simulink model "motor_io"  (Simulink 8.4)
settings: Solver=ode1  StartTime=0.0  StopTime=inf  FixedStep=Ts  RelTol=1e-3
PostLoadFcn:
  | , if any(exist('dsrtsu_mdlpostloadfcn', 'file') == [2, 3, 6]), try dsrtsu_mdlpostloadfcn('Execute', bdroot); catch fprintf('Error in PostLoadFcn (dsrtsu_mdlpostloadfcn) for model "%s":\n %s\n', bdroot, lasterr); end, end,
values from neighbouring files (symbols this model uses):
  enable_karnop = 1    [workshop1.m]
  F_c = 1e-3    (= 0.001)    [workshop1.m]
  J = J1+J2    (= 3.6e-05)    [workshop1.m]
  Jtot = motor.J + J/n^2    [workshop1.m]
  motor = motor_pars    [workshop1.m]
  n = 5    [workshop1.m]
  Ts = 0.02    [workshop1.m]
libraries: rtilib1104 x5, simulink x1
settings Model: DSRTSU_INTERNAL_RTI_VER=450  DSRTSU_INTERNAL_RTI_TYPE=rti1104  DSRTSU_INTERNAL_RTIFPGA=40  Creator=user  LastModifiedBy=es2lab2  ExtModeArmWhenConnect=off  BufferReuse=off
settings DataIOCC: SaveOutput=off  SignalLoggingName=sigsOut
settings OptimizationCC: BlockReduction=off  ConditionallyExecuteInputs=off  OptimizeBlockIOStorage=off  BufferReuse=off  GlobalBufferReuse=off  ExpressionFolding=off  LocalBlockOutputs=off  InitFltsAndDblsToZero=on
settings DebuggingCC: SaveWithParameterizedLinksMsg=none  SignalResolutionControl=TryResolveAllWithWarning  SolverPrmCheckMsg=none  MultiTaskDSMMsg=warning  MultiTaskCondExecSysMsg=none  UnconnectedInputMsg=none  UnconnectedOutputMsg=none
settings HardwareCC: ProdIntDivRoundTo=Zero  ProdEndianess=BigEndian  ProdHWDeviceType=Generic->Custom  TargetIntDivRoundTo=Zero  TargetEndianess=BigEndian  TargetHWDeviceType=Generic->Custom
settings RTWCC: SystemTargetFile=rti1104.tlc  MakeCommand=make_rti  TemplateMakefile=rti1104.tmf  Description=dSPACE DS1104 Hardware Platform  RetainRTWFile=on  ProcessScript=rti1104_make_rtw_hook  IncludeERTFirstTime=on
settings STFCustomTargetCC: TargetFcnLib=ansi_tfl_tmw.mat  ParMdlRefBuildCompliant=on  GeneratePreprocessorConditionals=Disable all  SystemTargetFile=rti1104.tlc
settings GRTTargetCC: TargetFcnLib=ansi_tfl_tmw.mat  CompOptLevelCompliant=off  ConcurrentExecutionCompliant=off  MatFileLogging=off  CPPClassGenCompliant=off  ExtModeMexFile=noextcomm
settings CustomProperty: DataType=RTWOptions_EnumType_C__Program Files (x86)_dSPACE RCPHIL 2014-B_MATLAB_RTI_RTI1104_TLC_rti1104_1InitialSimState  Value=RUN
settings EnumStrPairs: String=RUN

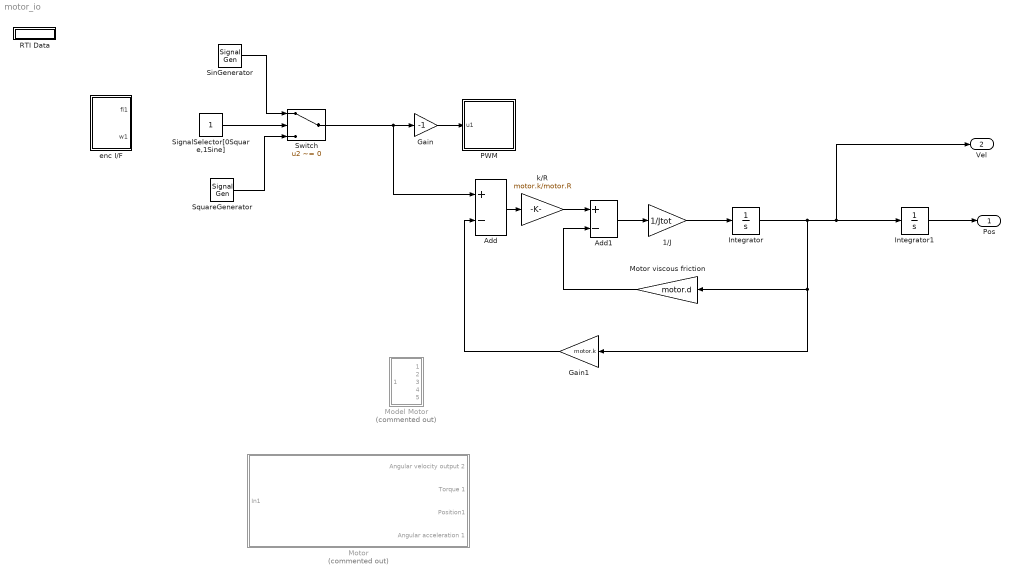
== system motor_io ==
  1/J : Gain  Gain=1/Jtot
  Add : Sum  Inputs=+-
  Add1 : Sum  Inputs=+-
  Gain : Gain  Gain=-1
  Gain1 : Gain  Gain=motor.k
  Integrator : Integrator
  Integrator1 : Integrator
  Model Motor : Subsystem  Commented=on
  Motor : Subsystem  Commented=on
  Motor viscous friction : Gain  Gain=motor.d
  PWM : Subsystem
  RTI Data : Subsystem  Tag=struct('RTIDataServer',struct('RTIDataServerVs','2','RTIModelDescription','struct(''main'',''motor_io'',''sub'','''',''isMp'',0)'))  LoadFcn="if exist('rtidc'), try,  rtidc('DataHostBlockClbLoad', gcbh); catch, disp(['Warning: ''LoadFcn'' for RTI Data block failed: ' lasterr]); end, end,"  mask(RTI_DATA_HOST){}
      mask help:
      | RTI Data Block.
      | This block is used by RTI to store internal model-dependent data.
      | Please keep this block on the root level of the model. Deleting this block will result in data loss.
      |
      | NEVER DELETE OR COPY THIS BLOCK!
      settings: CopyFcn="if exist('rtidc'), try,  rtidc('DataHostBlockClbCopy', gcbh); catch, disp(['Warning: ''CopyFcn'' for RTI Data block failed: ' lasterr]); end, end,"  DeleteFcn="if exist('rtidc'), try,  rtidc('DataHostBlockClbDelete', gcbh); catch, disp(['Warning: ''DeleteFcn'' for RTI Data block failed: ' lasterr]); end, end,"  ModelCloseFcn="if exist('rtidc'), try,  rtidc('DataHostBlockClbModelClose', gcbh); catch, disp(['Warning: ''ModelCloseFcn'' for RTI Data block failed: ' lasterr]); end, end,"  PreSaveFcn="if exist('rtidc'), try,  rtidc('DataHostBlockClbPreSave', gcbh); catch, disp(['Warning: ''PreSaveFcn'' for RTI Data block failed: ' lasterr]); end, end,"  PostSaveFcn="if exist('rtidc'), try,  rtidc('DataHostBlockClbPostSave', gcbh); catch, disp(['Warning: ''PostSaveFcn'' for RTI Data block failed: ' lasterr]); end, end,"  NameChangeFcn="if exist('rtidc'), try,  rtidc('DataHostBlockClbNameChange', gcbh); catch, disp(['Warning: ''NameChangeFcn'' for RTI Data block failed: ' lasterr]); end, end,"
      mask Help:
      | RTI Data Block.
      | This block is used by RTI to store internal model-dependent data.
      | Please keep this block on the root level of the model. Deleting this block will result in data loss.
      | 
      | NEVER DELETE OR COPY THIS BLOCK!
      mask Display:
      | text(0.5, 0.5, 'RTI Data', 'HorizontalAlignment', 'center');
      | plot([1 0]);
  SignalSelector[0Square,1Sine] : Constant
  SinGenerator : SignalGenerator  Amplitude=0  Units=rad/sec
  SquareGenerator : SignalGenerator  WaveForm=square  Amplitude=0  Units=rad/sec
  Switch : Switch  Criteria=u2 ~= 0
  enc I/F : Subsystem
  "k/R " : Gain  Gain=motor.k/motor.R
  Pos : Outport
  Vel : Outport  Port=2
  wires:
  SinGenerator/1 -> Switch/1
  SquareGenerator/1 -> Switch/3
  SignalSelector[0Square,1Sine]/1 -> Switch/2
  Switch/1 -> Add/1, Gain/1
  Gain1/1 -> Add/2
  Add/1 -> "k/R "/1
  "k/R "/1 -> Add1/1
  Add1/1 -> 1/J/1
  1/J/1 -> Integrator/1
  Integrator/1 -> Motor viscous friction/1, Gain1/1, Vel/1, Integrator1/1
  Motor viscous friction/1 -> Add1/2
  Integrator1/1 -> Pos/1
  Gain/1 -> PWM/1(u1)

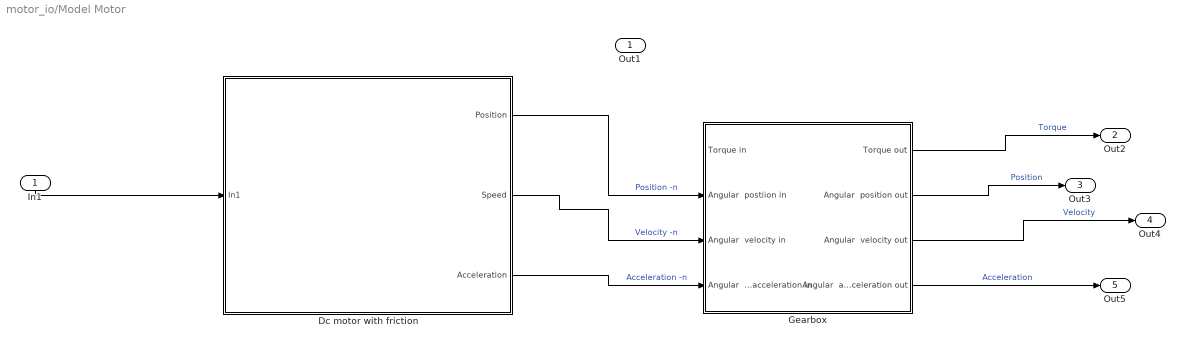
== system motor_io/Model Motor ==
  In1 : Inport
  Dc motor with friction : Subsystem
      mask Display:
      | image('dcmotor.jpg')
      | port_label('input', 1, 'Voltage')
      | port_label('output', 1, 'Current')
      | port_label('output', 2, 'Torque')
      | port_label('output', 3, 'Position')
      | port_label('output', 4, 'Velocity')
      | port_label('output', 5, 'Acceleration')
  Gearbox : Subsystem
  Out1 : Outport
  Out2 : Outport  Port=2
  Out3 : Outport  Port=3
  Out4 : Outport  Port=4
  Out5 : Outport  Port=5
  wires:
  Dc motor with friction/2(Speed) -> Gearbox/3(Angular  velocity in)  "Velocity -n"
  ? -> Gearbox/1(Torque in)  "Torque -n"
  Dc motor with friction/3(Acceleration) -> Gearbox/4(Angular  acceleration in)  "Acceleration -n"
  Dc motor with friction/1(Position) -> Gearbox/2(Angular  postiion in)  "Position -n"
  In1/1 -> Dc motor with friction/1(In1)
  Gearbox/1(Torque out) -> Out2/1  "Torque"
  ? -> Out1/1  "Current"
  Gearbox/2(Angular  position out) -> Out3/1  "Position"
  Gearbox/4(Angular  acceleration out) -> Out5/1  "Acceleration"
  Gearbox/3(Angular  velocity out) -> Out4/1  "Velocity"

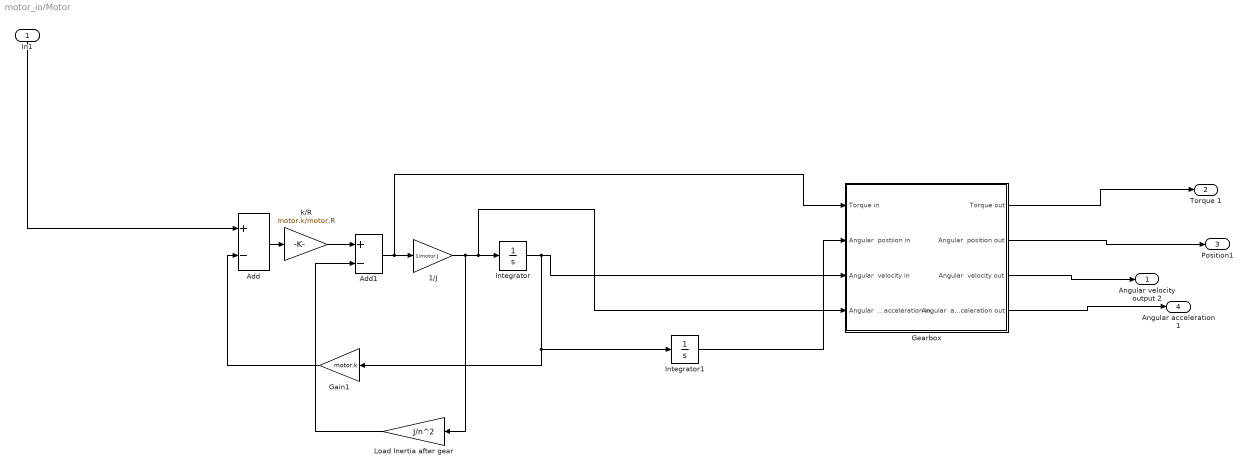
== system motor_io/Motor ==
  In1 : Inport
  1/J : Gain  Gain=1/motor.J
  Add : Sum  Inputs=+-
  Add1 : Sum  Inputs=+-
  Gain1 : Gain  Gain=motor.k
  Gearbox : Subsystem
  Integrator : Integrator
  Integrator1 : Integrator
  Load Inertia after gear : Gain  Gain=J/n^2
  "k/R " : Gain  Gain=motor.k/motor.R
  Angular velocity output 2 : Outport
  Torque 1 : Outport  Port=2
  Position1 : Outport  Port=3
  Angular acceleration 1 : Outport  Port=4
  wires:
  Integrator1/1 -> Gearbox/2(Angular  postiion in)
  Add/1 -> "k/R "/1
  "k/R "/1 -> Add1/1
  1/J/1 -> Load Inertia after gear/1, Gearbox/4(Angular  acceleration in), Integrator/1
  Add1/1 -> Gearbox/1(Torque in), 1/J/1
  Gain1/1 -> Add/2
  Integrator/1 -> Gearbox/3(Angular  velocity in), Integrator1/1, Gain1/1
  In1/1 -> Add/1
  Gearbox/4(Angular  acceleration out) -> Angular acceleration 1/1
  Gearbox/3(Angular  velocity out) -> Angular velocity output 2/1
  Gearbox/2(Angular  position out) -> Position1/1
  Gearbox/1(Torque out) -> Torque 1/1
  Load Inertia after gear/1 -> Add1/2

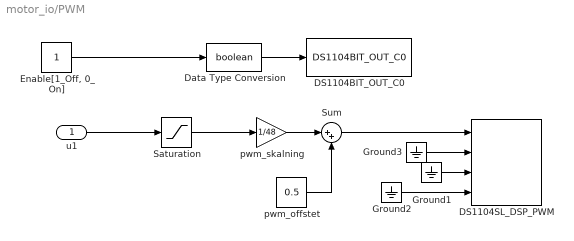
== system motor_io/PWM ==
  u1 : Inport
  DS1104BIT_OUT_C0 : rtilib1104/DS1104 MASTER PPC/DS1104BIT_OUT_C0  ChannelNo=0  InitValue=1  TermMode=0  TermValue=0  Reserved1=[]  Reserved2=[]  Reserved3=[]  Reserved=[]  DialogFcn=gui1104bit_out  UnitName={'DS1104BIT_OUT_C'}  UnitValues={ 0 }  DSProperties=struct('RTI',struct('Version',uint32(1),'BlockType',struct('isSLSource',uint8(0),'isSLSink',uint8(1),'isHWSource',uint8(0),'isHWSink',uint8(1),'isSetup',uint8(0),'isInline',uint8(1),'isNonInline',uint8(0),'isInterrupt',uint8(0),'isChannelwise',uint8(1)),'IOBoardType','DS1104MASTER','UnitType','BIT','Identifier','BITOUTCH','DialogType','ML','BlockSet','NONE','SlaveProcessor','NONE'))
  DS1104SL_DSP_PWM : rtilib1104/DS1104 SLAVE DSP/DS1104SL_DSP_PWM  Parameters=[]  TDef=[]  BoardType=[]  PwmMode=1  Frequency=20000  InitValue=[0.5 0.5 0.5 0.5]  TermMode=[0 0 0 0]  TermValue=[0.5 0.5 0.5 0.5]  Polarity=[1 1 1 1]  DialogFcn=gui1104sl_dsp_pwm  Reserved1=[]  Reserved2=[]  Reserved3=[]  Reserved4=[]  Revision=[]  UnitName={'DS1104SL_DSP_PWM'}  UnitValues={[]}  DSProperties=struct('RTI',struct('Version',uint32(2),'BlockType',struct('isSLSource',uint8(0),'isSLSink',uint8(1),'isHWSource',uint8(0),'isHWSink',uint8(1),'isSetup',uint8(0),'isInline',uint8(1),'isNonInline',uint8(0),'isInterrupt',uint8(0),'isChannelwise',uint8(0)),'IOBoardType','DS1104SLAVE','UnitType','PWM','Identifier','PWM','DialogType','ML','BlockSet','NONE','SlaveProcessor','F240'))  RTIBlockInterface=struct('InputPortsActive',[1 1 1 1],'InputPortsWidth',int32([1 1 1 1]),'InputPortsName',{{['PWM Channel 1'],['PWM Channel 2'],['PWM Channel 3'],['PWM Channel 4']}},'IWork',{{{'',uint32(4)}}},'DialogFcn','rti1104slavepwmgui','InitLevel',1,'BlockDisplay',{{'','auto'}},'IconTransparency','on','MultiSFcn',4,'BlockName',struct('Token',{{'DS1104SL_DSP_PWM'}}))  RTIBlockParameters=struct('PWMSymmetryMode',{{1,'OFF',[]}},'PWMFrequency',{{'50000','OFF',[]}},'PWMPolarityMode',{{[1 1 1 1 1],'OFF',[]}},'ChannelNo',{{[1 2 3 4],'OFF',[]}},'SuspendModeInit',{{[0 0 0 0 1],'OFF',[]}},'TTLModeInit',{{[2 2 2 2 2],'OFF',[]}},'DutyCycleInitValueCh1',{{'0.5','OFF',[]}},'DutyCycleInitValueCh2',{{'0.5','OFF',[]}},'DutyCycleInitValueCh3',{{'0.5','OFF',[]}},'DutyCycleInitValueCh4',{{'0.5','OFF',[]}},'DutyCycleInitValueCh5',{{'0.5','OFF',[]}},'EnablePWMStop',{{[0 0 0 0 0],'OFF',[]}},'SuspendModeTerm',{{[0 0 0 0 1],'OFF',[]}},'TTLModeTerm',{{[2 2 2 2 2],'OFF',[]}},'DutyCycleTermValueCh1',{{'0.5','OFF',[]}},'DutyCycleTermValueCh2',{{'0.5','OFF',[]}},'DutyCycleTermValueCh3',{{'0.5','OFF',[]}},'DutyCycleTermValueCh4',{{'0.5','OFF',[]}},'DutyCycleTermValueCh5',{{'0.5','OFF',[]}},'TLCFileName',{{'rti1104pwm','OFF',[]}})  RTISFcnParameters=struct('PWMSymmetryMode','double','PWMFrequency','double','PWMPolarityMode','double','ChannelNo','double','SuspendModeInit','double','TTLModeInit','double','DutyCycleInitValueCh1','double','DutyCycleInitValueCh2','double','DutyCycleInitValueCh3','double','DutyCycleInitValueCh4','double','EnablePWMStop','double','SuspendModeTerm','double','TTLModeTerm','double','DutyCycleTermValueCh1','double','DutyCycleTermValueCh2','double','DutyCycleTermValueCh3','double','DutyCycleTermValueCh4','double','TLCFileName','char')  RTIBlockParaDefault=struct('PWMSymmetryMode',1,'PWMFrequency',100,'PWMPolarityMode',[1 1 1 1 1],'ChannelNo',[1 2 3 4],'SuspendModeInit',[1 1 1 1 1],'TTLModeInit',[2 2 2 2 2],'DutyCycleInitValueCh1',0.5,'DutyCycleInitValueCh2',0.5,'DutyCycleInitValueCh3',0.5,'DutyCycleInitValueCh4',0.5,'DutyCycleInitValueCh5',0.5,'EnablePWMStop',[1 1 1 1 0],'SuspendModeTerm',[1 1 1 1 1],'TTLModeTerm',[2 2 2 2 2],'DutyCycleTermValueCh1',0.5,'DutyCycleTermValueCh2',0.5,'DutyCycleTermValueCh3',0.5,'DutyCycleTermValueCh4',0.5,'DutyCycleTermValueCh5',0.5,'TLCFileName','rti1104pwm')
  Data Type Conversion : DataTypeConversion  OutDataTypeStr=boolean  SaturateOnIntegerOverflow=on  RndMeth=Zero
  "Enable[1_Off, 0_On]" : Constant
  Ground1 : Ground
  Ground2 : Ground
  Ground3 : Ground
  Saturation : Saturate  UpperLimit=24  LowerLimit=-24
  Sum : Sum  Inputs=|++  SaturateOnIntegerOverflow=on
  pwm_offstet : Constant  Value=0.5
  pwm_skalning : Gain  Gain=1/48  SaturateOnIntegerOverflow=on  OutDataTypeStr=Inherit: Same as input  ParamDataTypeStr=Inherit: Same as input
  wires:
  "Enable[1_Off, 0_On]"/1 -> Data Type Conversion/1
  Data Type Conversion/1 -> DS1104BIT_OUT_C0/1
  pwm_skalning/1 -> Sum/1
  Sum/1 -> DS1104SL_DSP_PWM/1
  pwm_offstet/1 -> Sum/2
  u1/1 -> Saturation/1
  Ground1/1 -> DS1104SL_DSP_PWM/3
  Ground2/1 -> DS1104SL_DSP_PWM/4
  Ground3/1 -> DS1104SL_DSP_PWM/2
  Saturation/1 -> pwm_skalning/1

== system motor_io/RTI Data ==
  RTI Data Store : Subsystem  Tag="struct('public',struct('sub',struct('name',{{'motor_io'}},'data',{{struct('TH',struct('thTaskInfo',struct('taskType',{'TIMER','HWINT','TMRINT','SWINT','GLINT'},'tasksNumOf',{1,0,0,0,0},'srcIds',{{'TIMERA'},{},{},{},{}},'taskNames',{{['Timer Task 1']},{},{},{},{}})),'th_tc',struct('dataType','TASK','taskGroupId','','taskGroupList',{{}},'taskSchedulingPolicy','FCFS','taskType','TIMER','blkh',-1,'srcId','TIMERA','srcSgnName',['Timer A interrupt'],'srcCpuName','','taskName',['Timer Task 1  [0.02] s'],'taskNameDisplayExt','','smplTime',0.02,'smplTimeOffs',0,'hasFixedPriority',0,'priority',1,'hasFixedOvc',0,'ovcType',1,'ovcMax',1),'tc_th',struct('dataType','TASK','taskGroupId','','taskGroupList',{{}},'taskSchedulingPolicy','FCFS','taskType','TIMER','blkh',-1,'srcId','TIMERA','srcSgnName',['Timer A interrupt'],'srcCpuName','','taskName',['Timer Task 1  [0.02] s'],'taskNameDisplayExt','','smplTime',0.02,'smplTimeOffs',0,'hasFixedPriority',0,'priority',1,'hasFixedOvc',0,'ovcType',1,'ovcMax',1))}})),'private',struct('version',struct('dsVer',uint32(2)),'access',struct('modified',['04-Mar-2016 16:52:32'],'type','Model','isPerm',1)))"  mask(RTI_DATA_STORE){}
      mask help:
      | RTI Data Store Block. This block is used by RTI to store internal model dependent data. Deleting this block will result in data loss.
      |
      | NEVER DELETE, COPY, OR MODIFY THIS BLOCK!
      mask Help:
      | RTI Data Store Block. This block is used by RTI to store internal model dependent data. Deleting this block will result in data loss.
      | 
      | NEVER DELETE, COPY, OR MODIFY THIS BLOCK!
      mask Display: text(0.5, 0.5, ' ', 'HorizontalAlignment', 'center');

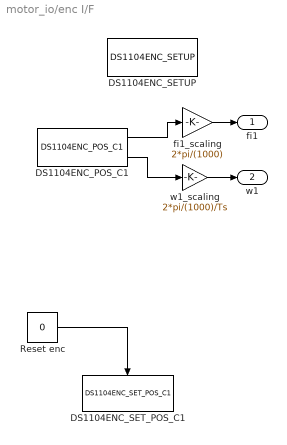
== system motor_io/enc I/F ==
  DS1104ENC_POS_C1 : rtilib1104/DS1104 MASTER PPC/DS1104ENC_POS_C1  ChannelNo=1  PosValue=0  Reserved1=[]  Reserved2=[]  Reserved3=[]  Reserved4=[]  DialogFcn=gui1104enc_pos  UnitName={'DS1104ENC_POS_C'}  UnitValues={ 1 }  DSProperties=struct('RTI',struct('Version',uint32(1),'BlockType',struct('isSLSource',uint8(1),'isSLSink',uint8(0),'isHWSource',uint8(1),'isHWSink',uint8(0),'isSetup',uint8(0),'isInline',uint8(1),'isNonInline',uint8(0),'isInterrupt',uint8(0),'isChannelwise',uint8(1)),'IOBoardType','DS1104MASTER','UnitType','ENC','Identifier','ENCPOSCH','DialogType','ML','BlockSet','NONE','SlaveProcessor','NONE'))
  DS1104ENC_SETUP : rtilib1104/DS1104 MASTER PPC/DS1104ENC_SETUP  Reserved1=[]  Reserved2=[]  Reserved3=[]  Reserved4=[]  DialogFcn=gui1104enc_setup  UnitName={'DS1104ENC_SETUP'}  UnitValues={ [] }  DSProperties=struct('RTI',struct('Version',uint32(1),'BlockType',struct('isSLSource',uint8(0),'isSLSink',uint8(0),'isHWSource',uint8(0),'isHWSink',uint8(0),'isSetup',uint8(0),'isInline',uint8(1),'isNonInline',uint8(0),'isInterrupt',uint8(0),'isChannelwise',uint8(0)),'IOBoardType','DS1104MASTER','UnitType','ENC','Identifier','ENCSETUP','DialogType','ML','BlockSet','NONE','SlaveProcessor','NONE'))
      settings: SignalType=[1 0]
  DS1104ENC_SET_POS_C1 : rtilib1104/DS1104 MASTER PPC/DS1104ENC_SET_POS_C1  ChannelNo=1  PosValue=0  Reserved1=[]  Reserved2=[]  Reserved3=[]  Reserved4=[]  DialogFcn=gui1104enc_set_pos  UnitName={'DS1104ENC_SET_POS_C'}  UnitValues={ 1 }  DSProperties=struct('RTI',struct('Version',uint32(1),'BlockType',struct('isSLSource',uint8(0),'isSLSink',uint8(1),'isHWSource',uint8(0),'isHWSink',uint8(1),'isSetup',uint8(0),'isInline',uint8(1),'isNonInline',uint8(0),'isInterrupt',uint8(0),'isChannelwise',uint8(1)),'IOBoardType','DS1104MASTER','UnitType','ENC','Identifier','ENCRESET','DialogType','ML','BlockSet','NONE','SlaveProcessor','NONE'))
  Reset enc : Constant  Value=0
  fi1_scaling : Gain  Gain=2*pi/(1000)  SaturateOnIntegerOverflow=on  OutDataTypeStr=Inherit: Same as input  ParamDataTypeStr=Inherit: Same as input
  w1_scaling : Gain  Gain=2*pi/(1000)/Ts  SaturateOnIntegerOverflow=on  OutDataTypeStr=Inherit: Same as input  ParamDataTypeStr=Inherit: Same as input
  fi1 : Outport
  w1 : Outport  Port=2
  wires:
  Reset enc/1 -> DS1104ENC_SET_POS_C1/Trigger
  DS1104ENC_POS_C1/1 -> fi1_scaling/1
  DS1104ENC_POS_C1/2 -> w1_scaling/1
  fi1_scaling/1 -> fi1/1
  w1_scaling/1 -> w1/1

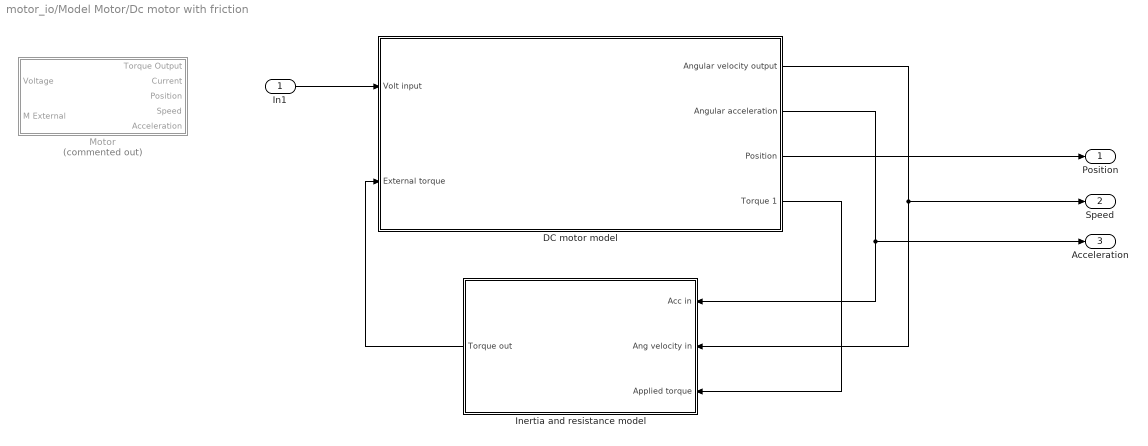
== system motor_io/Model Motor/Dc motor with friction ==
  In1 : Inport
  DC motor model : Subsystem
  "Inertia and resistance model " : Subsystem
  Motor : Subsystem  Commented=on
  Position : Outport
  Speed : Outport  Port=2
  Acceleration : Outport  Port=3
  wires:
  DC motor model/1("Angular velocity output ") -> "Inertia and resistance model "/2(Ang velocity in), Speed/1
  DC motor model/3(Position) -> Position/1
  In1/1 -> DC motor model/1("Volt input ")
  DC motor model/2("Angular acceleration ") -> "Inertia and resistance model "/1(Acc in), Acceleration/1
  "Inertia and resistance model "/1(Torque out) -> DC motor model/2(External torque)
  DC motor model/4(Torque 1) -> "Inertia and resistance model "/3(Applied torque)

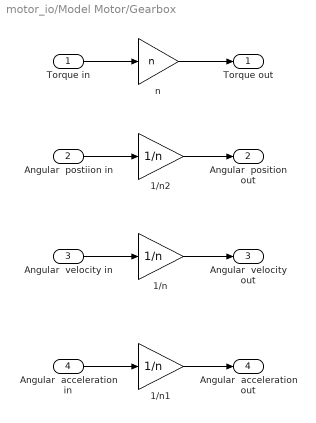
== system motor_io/Model Motor/Gearbox ==
  Torque in : Inport
  Angular  postiion in : Inport  Port=2
  Angular  velocity in : Inport  Port=3
  Angular  acceleration in : Inport  Port=4
  1/n : Gain  Gain=1/n
  1/n1 : Gain  Gain=1/n
  1/n2 : Gain  Gain=1/n
  n : Gain  Gain=n
  Torque out : Outport
  Angular  position out : Outport  Port=2
  Angular  velocity out : Outport  Port=3
  Angular  acceleration out : Outport  Port=4
  wires:
  1/n/1 -> Angular  velocity out/1
  Angular  velocity in/1 -> 1/n/1
  n/1 -> Torque out/1
  Torque in/1 -> n/1
  1/n1/1 -> Angular  acceleration out/1
  Angular  acceleration in/1 -> 1/n1/1
  1/n2/1 -> Angular  position out/1
  Angular  postiion in/1 -> 1/n2/1

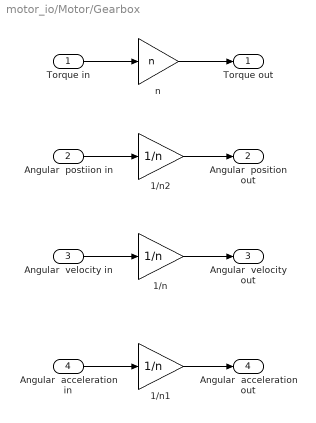
== system motor_io/Motor/Gearbox ==
  Torque in : Inport
  Angular  postiion in : Inport  Port=2
  Angular  velocity in : Inport  Port=3
  Angular  acceleration in : Inport  Port=4
  1/n : Gain  Gain=1/n
  1/n1 : Gain  Gain=1/n
  1/n2 : Gain  Gain=1/n
  n : Gain  Gain=n
  Torque out : Outport
  Angular  position out : Outport  Port=2
  Angular  velocity out : Outport  Port=3
  Angular  acceleration out : Outport  Port=4
  wires:
  1/n/1 -> Angular  velocity out/1
  Angular  velocity in/1 -> 1/n/1
  n/1 -> Torque out/1
  Torque in/1 -> n/1
  1/n1/1 -> Angular  acceleration out/1
  Angular  acceleration in/1 -> 1/n1/1
  1/n2/1 -> Angular  position out/1
  Angular  postiion in/1 -> 1/n2/1

== system motor_io/RTI Data/RTI Data Store ==
  RTI Data Store : Subsystem  mask(RTI_DATA_STORE){}
      mask help:
      | RTI Data Store Block. This block is used by RTI to store internal model dependent data. Deleting this block will result in data loss.
      |
      | NEVER DELETE, COPY, OR MODIFY THIS BLOCK!
      mask Help:
      | RTI Data Store Block. This block is used by RTI to store internal model dependent data. Deleting this block will result in data loss.
      | 
      | NEVER DELETE, COPY, OR MODIFY THIS BLOCK!
      mask Display: text(0.5, 0.5, ' ', 'HorizontalAlignment', 'center');

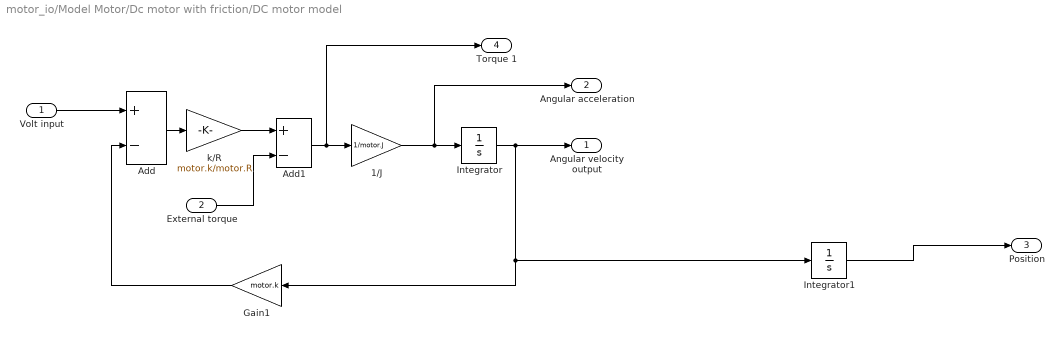
== system motor_io/Model Motor/Dc motor with friction/DC motor model ==
  "Volt input " : Inport
  External torque : Inport  Port=2
  1/J : Gain  Gain=1/motor.J
  Add : Sum  Inputs=+-
  Add1 : Sum  Inputs=+-
  Gain1 : Gain  Gain=motor.k
  Integrator : Integrator
  Integrator1 : Integrator
  "k/R " : Gain  Gain=motor.k/motor.R
  "Angular velocity output " : Outport
  "Angular acceleration " : Outport  Port=2
  Position : Outport  Port=3
  Torque 1 : Outport  Port=4
  wires:
  "Volt input "/1 -> Add/1
  Gain1/1 -> Add/2
  Add/1 -> "k/R "/1
  "k/R "/1 -> Add1/1
  Add1/1 -> Torque 1/1, 1/J/1
  1/J/1 -> "Angular acceleration "/1, Integrator/1
  Integrator/1 -> Integrator1/1, Gain1/1, "Angular velocity output "/1
  External torque/1 -> Add1/2
  Integrator1/1 -> Position/1

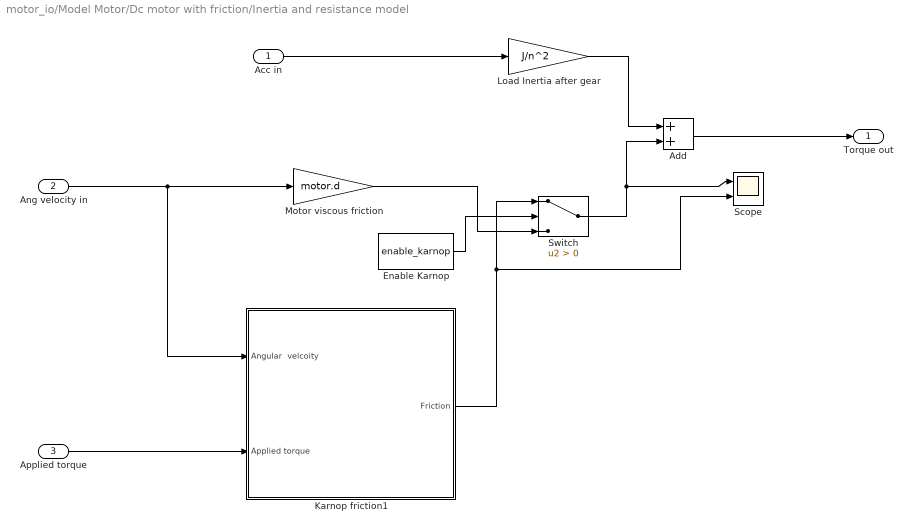
== system motor_io/Model Motor/Dc motor with friction/Inertia and resistance model  ==
  Acc in : Inport
  Ang velocity in : Inport  Port=2
  Applied torque : Inport  Port=3
  Add : Sum
  Enable Karnop : Constant  Value=enable_karnop
  Karnop friction1 : Subsystem
  Load Inertia after gear : Gain  Gain=J/n^2
  Motor viscous friction : Gain  Gain=motor.d
  Scope : Scope  NumInputPorts=2
      settings: YMin=-0.00177~-0.00177  YMax=0.00177~0.00177
  Switch : Switch  Criteria=u2 > Threshold
  Torque out : Outport
  wires:
  Add/1 -> Torque out/1
  Ang velocity in/1 -> Karnop friction1/1(Angular  velcoity), Motor viscous friction/1
  Motor viscous friction/1 -> Switch/3
  Karnop friction1/1(Friction) -> Switch/1, Scope/2
  Switch/1 -> Add/2, Scope/1
  Enable Karnop/1 -> Switch/2
  Applied torque/1 -> Karnop friction1/2("Applied torque ")
  Acc in/1 -> Load Inertia after gear/1
  Load Inertia after gear/1 -> Add/1

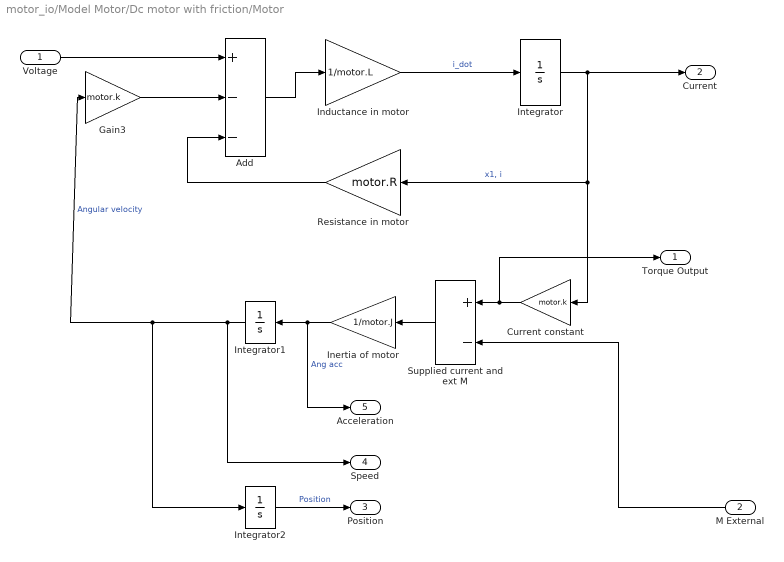
== system motor_io/Model Motor/Dc motor with friction/Motor ==
  Voltage : Inport
  "M External " : Inport  Port=2
  Add : Sum  Inputs=+--
  Current constant : Gain  Gain=motor.k
  Gain3 : Gain  Gain=motor.k
  Inductance in motor : Gain  Gain=1/motor.L
  Inertia of motor : Gain  Gain=1/motor.J
  Integrator : Integrator
  Integrator1 : Integrator
  Integrator2 : Integrator
  Resistance in motor : Gain  Gain=motor.R
  "Supplied current and ext M " : Sum  Inputs=+-
  Torque Output : Outport
  Current : Outport  Port=2
  Position : Outport  Port=3
  Speed : Outport  Port=4
  Acceleration : Outport  Port=5
  wires:
  Voltage/1 -> Add/1
  Add/1 -> Inductance in motor/1
  Inductance in motor/1 -> Integrator/1  "i_dot"
  Integrator/1 -> Current constant/1, Resistance in motor/1, Current/1  "x1, i"
  Resistance in motor/1 -> Add/3
  Gain3/1 -> Add/2
  Integrator1/1 -> Speed/1, Integrator2/1, Gain3/1  "Angular velocity"
  "Supplied current and ext M "/1 -> Inertia of motor/1
  Inertia of motor/1 -> Acceleration/1, Integrator1/1  "Ang acc"
  Current constant/1 -> Torque Output/1, "Supplied current and ext M "/1
  "M External "/1 -> "Supplied current and ext M "/2
  Integrator2/1 -> Position/1  "Position"

== system motor_io/RTI Data/RTI Data Store/RTI Data Store ==
  RTI Data Store : Subsystem  mask(RTI_DATA_STORE){}
      mask help:
      | RTI Data Store Block. This block is used by RTI to store internal model dependent data. Deleting this block will result in data loss.
      |
      | NEVER DELETE, COPY, OR MODIFY THIS BLOCK!
      mask Help:
      | RTI Data Store Block. This block is used by RTI to store internal model dependent data. Deleting this block will result in data loss.
      | 
      | NEVER DELETE, COPY, OR MODIFY THIS BLOCK!
      mask Display: text(0.5, 0.5, ' ', 'HorizontalAlignment', 'center');

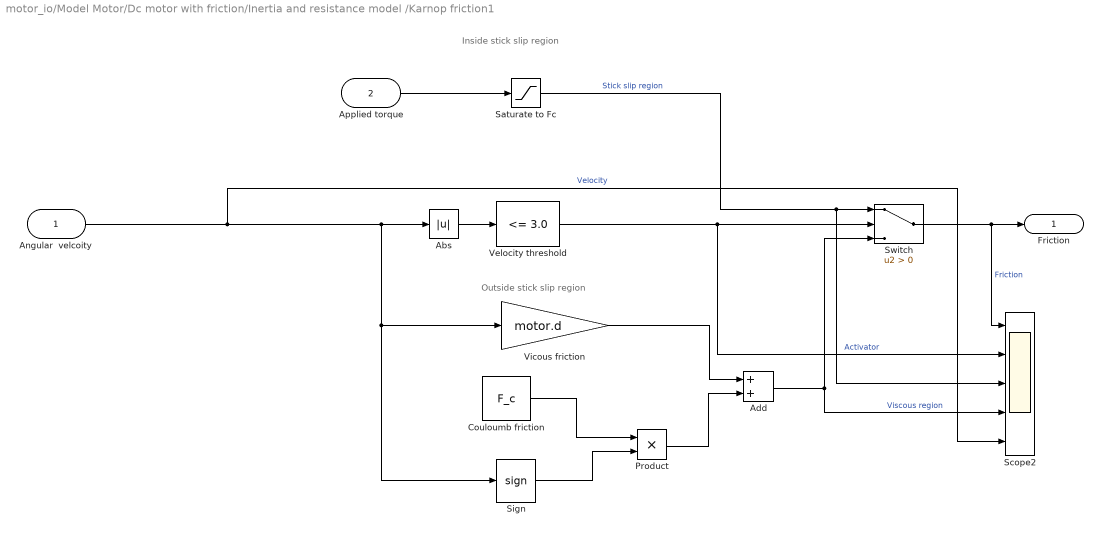
== system motor_io/Model Motor/Dc motor with friction/Inertia and resistance model /Karnop friction1 ==
  note: Inside stick slip region
  note: Outside stick slip region
  Angular  velcoity : Inport
  "Applied torque " : Inport  Port=2
  Abs : Abs
  Add : Sum
  Couloumb friction : Constant  Value=F_c
  Product : Product
  Saturate to Fc : Saturate  UpperLimit=F_c  LowerLimit=-F_c
  Scope2 : Scope  NumInputPorts=5
      settings: ShowLegends=on  YMin=-0.00177~-0.125~0.0009~-0.00177~-138.1533~-0.12501~-0.12501~-0.12501  YMax=0.00177~1.125~0.0011~0.00177~138.10681~0.12501~0.12501~0.12501  SaveName=ScopeData3
  Sign : Signum
  Switch : Switch  Criteria=u2 > Threshold
  "Velocity threshold " : simulink/Logic and Bit Operations/Compare To Constant  relop=<=  const=3.0  OutDataTypeStr=boolean
  Vicous friction : Gain  Gain=motor.d
  Friction : Outport
  wires:
  Saturate to Fc/1 -> Scope2/3, Switch/1  "Stick slip region"
  Switch/1 -> Scope2/1, Friction/1  "Friction"
  Angular  velcoity/1 -> Scope2/5, Abs/1, Vicous friction/1, Sign/1  "Velocity"
  "Velocity threshold "/1 -> Scope2/2, Switch/2  "Activator"
  Abs/1 -> "Velocity threshold "/1
  Product/1 -> Add/2
  Vicous friction/1 -> Add/1
  Couloumb friction/1 -> Product/1
  Sign/1 -> Product/2
  "Applied torque "/1 -> Saturate to Fc/1
  Add/1 -> Switch/3, Scope2/4  "Viscous region"

== system motor_io/RTI Data/RTI Data Store/RTI Data Store/RTI Data Store ==
  RTI Data Store : Subsystem  mask(RTI_DATA_STORE){}
      mask help:
      | RTI Data Store Block. This block is used by RTI to store internal model dependent data. Deleting this block will result in data loss.
      |
      | NEVER DELETE, COPY, OR MODIFY THIS BLOCK!
      mask Help:
      | RTI Data Store Block. This block is used by RTI to store internal model dependent data. Deleting this block will result in data loss.
      | 
      | NEVER DELETE, COPY, OR MODIFY THIS BLOCK!
      mask Display: text(0.5, 0.5, ' ', 'HorizontalAlignment', 'center');

== system motor_io/RTI Data/RTI Data Store/RTI Data Store/RTI Data Store/RTI Data Store ==
